simulink model "Adder_Multiplier"  (R2021b)
settings: Solver=VariableStepAuto  StartTime=0.0  StopTime=10.0  RelTol=1e-3
settings Model: Creator=Student  LastModifiedBy=Student

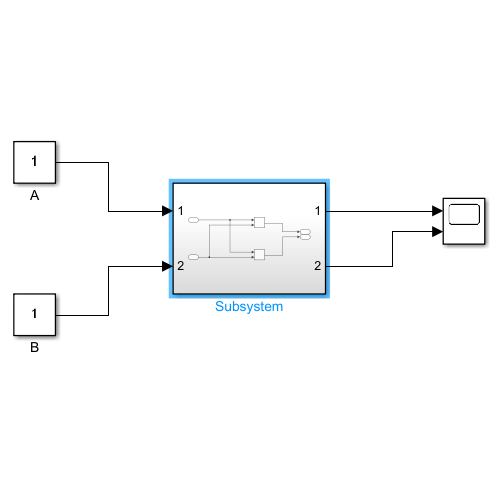
[thumbnail: Simulink's stored preview of the top-level diagram]
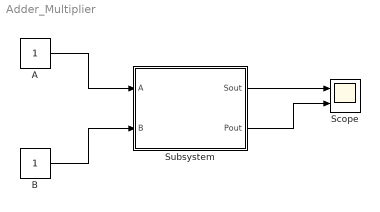
== system Adder_Multiplier ==
  A : Constant  SampleTime=-1
  B : Constant  SampleTime=-1
  Scope : Scope  NumInputPorts=2
  Subsystem : Subsystem
  wires:
  A/1 -> Subsystem/1(A)
  B/1 -> Subsystem/2(B)
  Subsystem/1(Sout) -> Scope/1
  Subsystem/2(Pout) -> Scope/2

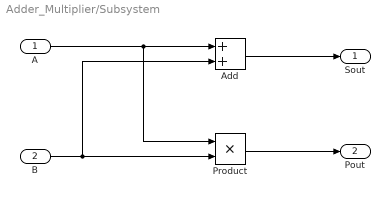
== system Adder_Multiplier/Subsystem ==
  A : Inport
  B : Inport  Port=2
  Add : Sum
  Product : Product
  Sout : Outport
  Pout : Outport  Port=2
  wires:
  B/1 -> Add/2, Product/2
  A/1 -> Product/1, Add/1
  Add/1 -> Sout/1
  Product/1 -> Pout/1
